simulink model "hiperman_4_2007b_FixPt"  (Simulink 7.2)
settings: Solver=VariableStepDiscrete  SolverMode=SingleTasking  StartTime=0.0  StopTime=inf  RelTol=1e-3
PreLoadFcn:
  | SNR = 17;
  | wl = 16;
undefined symbols (not defined in the file or in its folder): Deinterleaver, get, hiperman_lib, Interleaver
libraries: commutil2 x7, dspobslib x5, commblkcod2 x3, dspsigops x3, commdigbbndam3 x2, commblkintrlv2 x2, dspindex x2, commsequence2 x2, commcnvcod2 x2, commsink2 x2, dspmtrx3 x2, commchan3 x1
CloseFcn:
  | rtwprivate ssgencode ModelCloseRequest hiperman_4_2007b_FixPt
settings Model: Creator=mikem  LastModifiedBy=mdonovan
settings DataIOCC: SaveOutput=off  SaveTime=off
settings OptimizationCC: InlineParams=on  InlineInvariantSignals=on  EnforceIntegerDowncast=off  StateBitsets=on  DataBitsets=on  UseTempVars=on  ZeroExternalMemoryAtStartup=off  ZeroInternalMemoryAtStartup=off  OptimizeModelRefInitCode=on  LifeSpan=1
settings DebuggingCC: AlgebraicLoopMsg=error  SaveWithParameterizedLinksMsg=none  SignalResolutionControl=TryResolveAllWithWarning  MultiTaskDSMMsg=warning  MultiTaskCondExecSysMsg=none  SingleTaskRateTransMsg=error  StrictBusMsg=None  LoggingUnavailableSignals=none
settings HardwareCC: ProdHWDeviceType=Generic->32-bit Embedded Processor  TargetHWDeviceType=32-bit Generic  ProdEqTarget=off
settings RTWCC: SystemTargetFile=ert.tlc  GenCodeOnly=on  TemplateMakefile=ert_default_tmf  Description=Real-Time Workshop Embedded Coder (no auto configuration)  GenerateReport=on  ProcessScript=ert_make_rtw_hook  IncludeHyperlinkInReport=on  LaunchReport=on  IncludeERTFirstTime=on
settings CodeAppCC: IgnoreCustomStorageClasses=off
settings ERTTargetCC: MultiwordLength=2048  GenerateSampleERTMain=on  InlinedParameterPlacement=NonHierarchical  ERTCustomFileTemplate=example_file_process.tlc

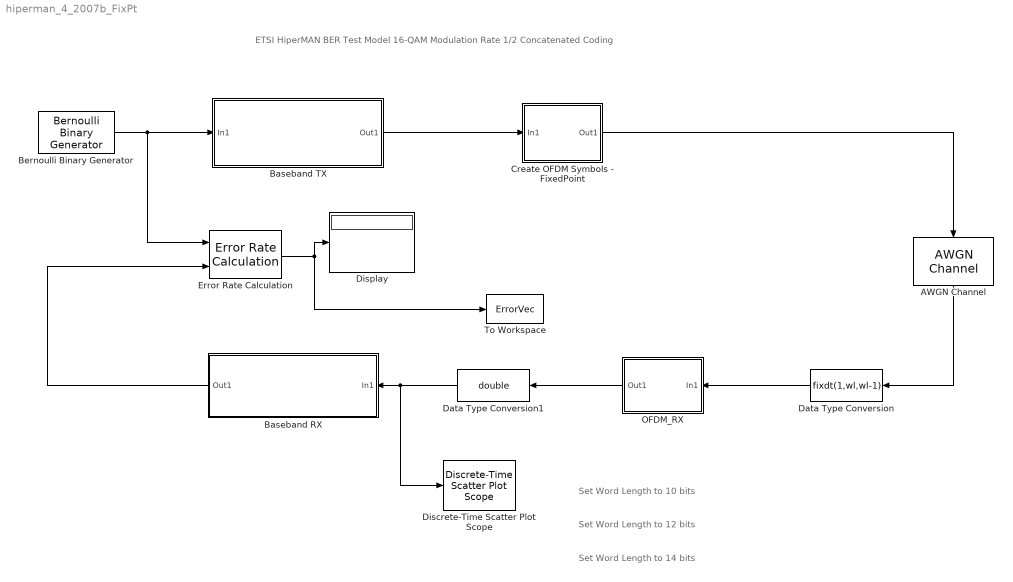
== system hiperman_4_2007b_FixPt ==
  note: ETSI HiperMAN
      | BER Test Model
      | 16-QAM Modulation
      | Rate 1/2 Concatenated Coding
  note: Set Word Length to 12 bits
  note: Set Word Length to 14 bits
  note: Set Word Length to 10 bits
  AWGN Channel : commchan3/AWGN Channel  Orientation=down  SystemSampleTime=-1  seed=67  noiseMode="Signal to noise ratio  (SNR)"  EbNodB=10  EsNodB=10  SNRdB=SNR  bitsPerSym=1  Ps=2/192  Tsym=1  variance=.0004
  Baseband RX : Subsystem  Orientation=left
  Baseband TX : Subsystem
  Bernoulli Binary Generator : commrandsrc2/Bernoulli Binary Generator  DialogController=commDDGCreate  DialogControllerArgs=DataTag3  SystemSampleTime=-1  P=0.5  seed=61  Ts=864/(20e6*3/4*6*32/33*3/4*8/7)/384  frameBased=on  sampPerFrame=384  orient=off  outDataType=double
  Create OFDM Symbols - FixedPoint : Subsystem
      mask Display: disp('Create OFDM\nSymbols');
  Data Type Conversion : DataTypeConversion  Orientation=left  OutDataTypeMode=Specify via dialog  OutDataType=fixdt(1,wl,wl-1)  OutDataTypeStr=fixdt(1,wl,wl-1)
  Data Type Conversion1 : DataTypeConversion  Orientation=left  OutDataTypeMode=double  OutDataType=fixdt(1,16,12)  OutDataTypeStr=double
  Discrete-Time Scatter Plot Scope : commsink2/Discrete-Time Scatter Plot Scope  Tag=ScatterPlot  SystemSampleTime=-1  sampPerSymb=1  offsetEye=0  numTraces=384  numNewFrames=384  LineMarkers=.  LineColors=b  fading=on  render=on  AxisGrid=on  xMin=-1.57265625  xMax=1.47890625  yMin=-1.61953125  yMax=1.43203125  inphaseLabel=In-phase Amplitude  quadratureLabel=Quadrature Amplitude  openScopeAtSimStart=on  FrameNumber=off  FigPos=get(0,'defaultfigureposition');  figTitle=Scatter Plot  numLinesMax=8  block_type_=scatter
  Display : Display
  Error Rate Calculation : commsink2/Error Rate Calculation  N=0  st_delay=0  cp_mode=Entire frame  subframe=[]  PMode=Port  WsName=ErrorVec  RsMode2=off  stop=on  numErr=100  maxBits=1e6
  OFDM_RX : Subsystem  Orientation=left  MinMaxOverflowLogging=MinMaxAndOverflow
      mask Display: disp('Extract Data\nSymbols');
  To Workspace : ToWorkspace  VariableName=ErrorVec  SampleTime=-1  SaveFormat=Array
      settings: MaxDataPoints=1
  wires:
  Create OFDM Symbols - FixedPoint/1(Out1) -> AWGN Channel/1
  AWGN Channel/1 -> Data Type Conversion/1
  Baseband RX/1(Out1) -> Error Rate Calculation/2
  Bernoulli Binary Generator/1 -> Error Rate Calculation/1, Baseband TX/1(In1)
  Baseband TX/1(Out1) -> Create OFDM Symbols - FixedPoint/1(In1)
  Error Rate Calculation/1 -> Display/1, To Workspace/1
  OFDM_RX/1(Out1) -> Data Type Conversion1/1
  Data Type Conversion/1 -> OFDM_RX/1(In1)
  Data Type Conversion1/1 -> Baseband RX/1(In1), Discrete-Time Scatter Plot Scope/1

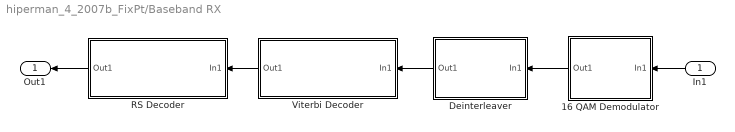
== system hiperman_4_2007b_FixPt/Baseband RX ==
  In1 : Inport  Orientation=left
  16 QAM Demodulator : Subsystem  Orientation=left  AncestorBlock=hiperman_lib/16 QAM Demodulator
      mask init:
      | Ry = ones(4,1)*[+1 +3 -1 -3];
      | Iy = [+1 +3 -3 -1]'*ones(1,4);
      | qamConst = Ry+j*Iy;
      | qamConst = qamConst(:)/sqrt(10);
      | clear Ry Iy;
      mask Display: disp('16 QAM\nDemodulator')
  Deinterleaver : Subsystem  Orientation=left  AncestorBlock=hiperman_lib/Deinterleaver  mask{n1=768, n2=4}
      mask prompts: n1 "Number of coded bits per subchannel:"; n2 "Number of coded bits per subcarrier:"
      mask init:
      | bpc = [192 384 768 1152];
      | pc = [1 2 4 6];
      | Ncbps = bpc(n1);
      | Ncpc = pc(n2);
      | 
      | k = 0:Ncbps-1;
      | mk = (Ncbps/12)*mod(k,12)+floor(k/12);
      | 
      | s = ceil(Ncpc/2);
      | jk = s*floor(mk/s)+mod(mk+Ncbps-floor(12*mk/Ncbps),s);
      | 
      | [x,int_idx] = sort(jk);
      | 
      | clear bpc pc Ncbps Ncpc k mk s jk x
      mask StyleString: popup(192|384|768|1152),popup(1|2|4|6)
      mask Display: disp('Deinterleaver');
  RS Decoder : Subsystem  Orientation=left  AncestorBlock=hiperman_lib/RS Decoder  mask{N=64, K=48}
      mask prompts: N "Input block size (N):"; K "Output block size (K):"
      mask init:
      | % The primitive polynomial is defined over GF(2)
      | primPoly = [1 0 0 0 1 1 1 0 1];  
      | % The generator polynomial is defined over GF(2^8)
      | genPoly = gf([1 1],8);
      | for idx = 1:15
      |     genPoly = conv(genPoly,[1 gf(2,8)^idx]);
      | end
      mask Display: disp('Shortened and Punctured\nReed-Solomon Decoder')
  Viterbi Decoder : Subsystem  Orientation=left  AncestorBlock=hiperman_lib/Viterbi Decoder  mask{ppat=[1 1 0 1]}
      mask prompts: ppat "Puncture pattern:"
      mask Display: disp('Viterbi Decoder\nfor Punctured\nConvolutional Code');
  Out1 : Outport  Orientation=left
  wires:
  16 QAM Demodulator/1(Out1) -> Deinterleaver/1(In1)
  Viterbi Decoder/1(Out1) -> RS Decoder/1(In1)
  Deinterleaver/1(Out1) -> Viterbi Decoder/1(In1)
  In1/1 -> 16 QAM Demodulator/1(In1)
  RS Decoder/1(Out1) -> Out1/1

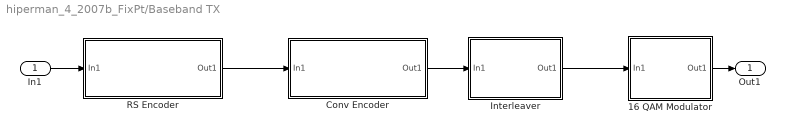
== system hiperman_4_2007b_FixPt/Baseband TX ==
  In1 : Inport
  16 QAM Modulator : Subsystem  AncestorBlock=hiperman_lib/16 QAM Modulator
      mask init:
      | Ry = ones(4,1)*[+1 +3 -1 -3];
      | Iy = [+1 +3 -3 -1]'*ones(1,4);
      | qamConst = Ry+j*Iy;
      | qamConst = qamConst(:)/sqrt(10);
      | clear Ry Iy;
      mask Display: disp('16 QAM\nModulator');
  Conv Encoder : Subsystem  AncestorBlock=hiperman_lib/Conv Encoder  mask{ppat=[1 1 0 1]}
      mask prompts: ppat "Puncture pattern:"
      mask Display: disp('Punctured\nConvolutional Code');
  Interleaver : Subsystem  AncestorBlock=hiperman_lib/Interleaver  mask{n1=768, n2=4}
      mask prompts: n1 "Number of coded bits per subchannel:"; n2 "Number of coded bits per subcarrier:"
      mask init: same as hiperman_4_2007b_FixPt/Baseband RX/Deinterleaver
      mask StyleString: popup(192|384|768|1152),popup(1|2|4|6)
      mask Display: disp('Interleaver')
  RS Encoder : Subsystem  RequirementInfo={'other' 'D:\MBDC2005\ts_102177v010201p.pdf' '#12' 'true' 'Reed-Solomon Coding' '' } %GIDa_a12e56f2_2c6a_45c7_812c_df811bfc8a20  AncestorBlock=hiperman_lib/RS Encoder  mask{N=64, K=48}
      mask prompts: N "Output block size (N):"; K "Input block size (K):"
      mask init: same as hiperman_4_2007b_FixPt/Baseband RX/RS Decoder
      mask Display: disp('Shortened and Punctured\nReed-Solomon Encoder')
  Out1 : Outport
  wires:
  RS Encoder/1(Out1) -> Conv Encoder/1(In1)
  Conv Encoder/1(Out1) -> Interleaver/1(In1)
  Interleaver/1(Out1) -> 16 QAM Modulator/1(In1)
  In1/1 -> RS Encoder/1(In1)
  16 QAM Modulator/1(Out1) -> Out1/1

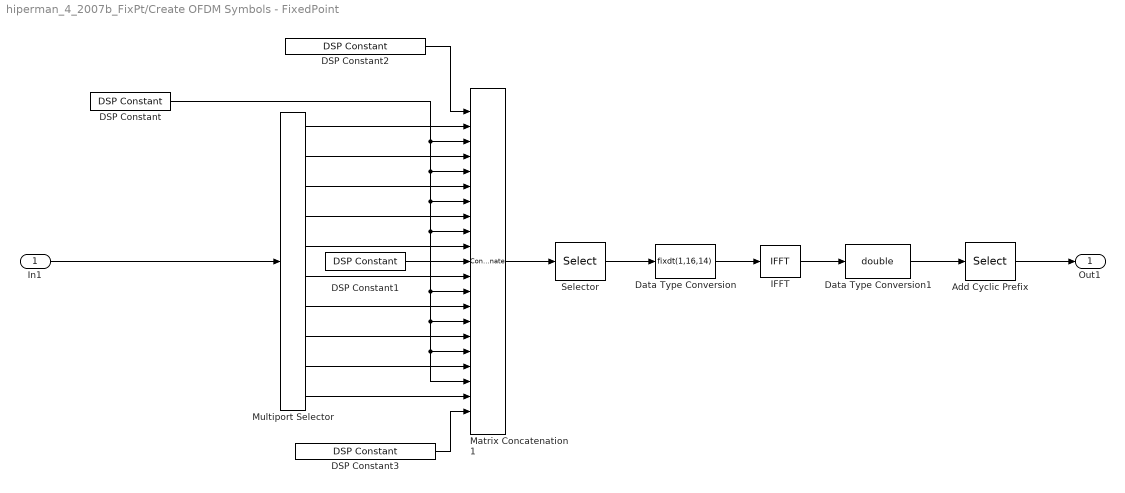
== system hiperman_4_2007b_FixPt/Create OFDM Symbols - FixedPoint ==
  In1 : Inport  OutDataType=sfix(16)  OutScaling=2^0
  Add Cyclic Prefix : Selector  NumberOfDimensions=2  InputPortWidth=3  IndexOptions=Index vector (dialog),Index vector (dialog)  Indices=[251:256 1:256],1  OutputSizes=1,1
  DSP Constant : dspobslib/DSP Constant  SystemSampleTime=-1  Value=complex(1,0)  SampleMode=Discrete  discreteOutput=Frame-based  continuousOutput=Sample-based  sampTime=1  framePeriod=inf  dataType=Inherit from 'Constant value'  isSigned=on  wordLen=16  udDataType=sfix(16)  fracBitsMode=Best precision  numFracBits=15  InterpretAs1D=-inf  Ts=-inf  FramebasedOutput=-inf
  DSP Constant1 : dspobslib/DSP Constant  SystemSampleTime=-1  Value=complex(0,0)  SampleMode=Discrete  discreteOutput=Frame-based  continuousOutput=Sample-based  sampTime=1  framePeriod=inf  dataType=Inherit from 'Constant value'  isSigned=on  wordLen=16  udDataType=sfix(16)  fracBitsMode=Best precision  numFracBits=15  InterpretAs1D=-inf  Ts=-inf  FramebasedOutput=-inf
  DSP Constant2 : dspobslib/DSP Constant  SystemSampleTime=-1  Value=complex(0,0)*ones(28,1)  SampleMode=Discrete  discreteOutput=Frame-based  continuousOutput=Sample-based  sampTime=1  framePeriod=inf  dataType=Inherit from 'Constant value'  isSigned=on  wordLen=16  udDataType=sfix(16)  fracBitsMode=Best precision  numFracBits=15  InterpretAs1D=-inf  Ts=-inf  FramebasedOutput=-inf
  DSP Constant3 : dspobslib/DSP Constant  SystemSampleTime=-1  Value=complex(0,0)*ones(27,1)  SampleMode=Discrete  discreteOutput=Frame-based  continuousOutput=Sample-based  sampTime=1  framePeriod=inf  dataType=Inherit from 'Constant value'  isSigned=on  wordLen=16  udDataType=sfix(16)  fracBitsMode=Best precision  numFracBits=15  InterpretAs1D=-inf  Ts=-inf  FramebasedOutput=-inf
  Data Type Conversion : DataTypeConversion  OutDataTypeMode=Specify via dialog  OutDataType=fixdt(1,16,14)  OutDataTypeStr=fixdt(1,16,14)
  Data Type Conversion1 : DataTypeConversion  OutDataTypeMode=double  OutDataType=fixdt(1,16,12)  OutDataTypeStr=double
  IFFT : dspxfrm3/IFFT  DialogController=dspDDGCreate  DialogControllerArgs=DataTag4  CompMethod=Table lookup  TableOpt=HYBRID  TableOptActive=Speed  BitRevOrder=off  cs_in=off  SkipNorm=on  InheritFFTLength=on  FFTLength=64  mode=Complex  outSamplingMode=Frame based  outputMode=Binary point scaling  outputWordLength=16  outputFracLength=14  accumMode=Binary point scaling  accumWordLength=32  accumFracLength=29  prodOutputMode=Binary point scaling  prodOutputWordLength=32  prodOutputFracLength=30  roundingMode=Floor  overflowMode=off
  Matrix Concatenation1 : Concatenate  NumInputs=21  Mode=Multidimensional array
  Multiport Selector : dspindex/Multiport Selector  rowsOrCols=Rows  idxCellArray={[1:12],[13:36],[37:60],[61:84],[85:96],[97:108],[109:132],[133:156],[157:180],[181:192]}  idxErrMode=Generate Error
  Selector : Selector  InputPortWidth=256  IndexOptions=Index vector (dialog)  Indices=[129:256 1:128]  OutputSizes=1
  Out1 : Outport  OutDataType=sfix(16)  OutScaling=2^0
  wires:
  Data Type Conversion1/1 -> Add Cyclic Prefix/1
  Data Type Conversion/1 -> IFFT/1
  DSP Constant/1 -> Matrix Concatenation1/3, Matrix Concatenation1/5, Matrix Concatenation1/7, Matrix Concatenation1/9, Matrix Concatenation1/13, Matrix Concatenation1/15, Matrix Concatenation1/17, Matrix Concatenation1/19
  Multiport Selector/10 -> Matrix Concatenation1/20
  Multiport Selector/9 -> Matrix Concatenation1/18
  Multiport Selector/8 -> Matrix Concatenation1/16
  Multiport Selector/7 -> Matrix Concatenation1/14
  Multiport Selector/6 -> Matrix Concatenation1/12
  Multiport Selector/5 -> Matrix Concatenation1/10
  Multiport Selector/4 -> Matrix Concatenation1/8
  Multiport Selector/3 -> Matrix Concatenation1/6
  Multiport Selector/2 -> Matrix Concatenation1/4
  Multiport Selector/1 -> Matrix Concatenation1/2
  DSP Constant1/1 -> Matrix Concatenation1/11
  DSP Constant2/1 -> Matrix Concatenation1/1
  DSP Constant3/1 -> Matrix Concatenation1/21
  Matrix Concatenation1/1 -> Selector/1
  In1/1 -> Multiport Selector/1
  Selector/1 -> Data Type Conversion/1
  IFFT/1 -> Data Type Conversion1/1
  Add Cyclic Prefix/1 -> Out1/1

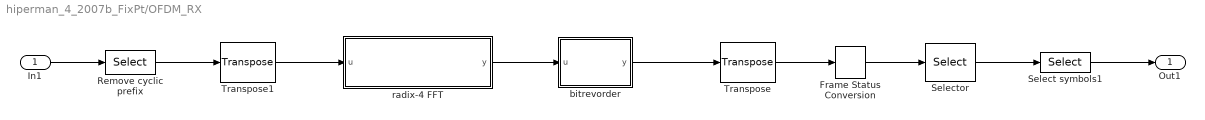
== system hiperman_4_2007b_FixPt/OFDM_RX ==
  In1 : Inport  OutDataType=sfix(16)  OutScaling=2^0
  Frame Status Conversion : dspobslib/Frame Status Conversion  SystemSampleTime=-1  growRefPort=off  outframe=Frame-based
  Remove cyclic prefix : Selector  NumberOfDimensions=2  InputPortWidth=80  IndexOptions=Index vector (dialog),Select all  Indices=[7:262],-1  OutputSizes=1
  Select symbols1 : Selector  NumberOfDimensions=2  InputPortWidth=64  IndexOptions=Index vector (dialog),Select all  Indices=[29:40 42:65 67:90 92:115 117:128 130:141 143:166 168:191 193:216 218:229],-1  OutputSizes=1
  Selector : Selector  InputPortWidth=256  IndexOptions=Index vector (dialog)  Indices=[129:256 1:128]  OutputSizes=1
  Transpose : dspmtrx3/Transpose  SystemSampleTime=-1  Hermitian=off  overflowFlag=off
  Transpose1 : dspmtrx3/Transpose  SystemSampleTime=-1  Hermitian=off  overflowFlag=off
  bitrevorder : Stateflow chart
  radix-4 FFT : Stateflow chart
  Out1 : Outport  OutDataType=sfix(16)  OutScaling=2^0
  wires:
  Transpose1/1 -> radix-4 FFT/1(u)
  Transpose/1 -> Frame Status Conversion/1
  radix-4 FFT/1(y) -> bitrevorder/1(u)
  Remove cyclic prefix/1 -> Transpose1/1
  Frame Status Conversion/1 -> Selector/1
  Selector/1 -> Select symbols1/1
  In1/1 -> Remove cyclic prefix/1
  Select symbols1/1 -> Out1/1
  bitrevorder/1(y) -> Transpose/1

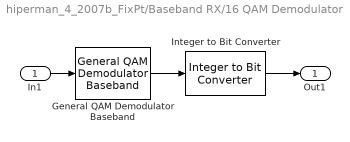
== system hiperman_4_2007b_FixPt/Baseband RX/16 QAM Demodulator ==
  In1 : Inport  OutDataType=sfix(16)  OutScaling=2^0
  General QAM Demodulator Baseband : commdigbbndam3/General QAM Demodulator Baseband  DialogController=commDDGCreate  DialogControllerArgs=DataTag0  SigCon=qamConst  OutType=Integer  DecType=Hard decision  VarSource=Dialog  Variance=1  outDtypeBit=Inherit via internal rule  outDtype=double  roundingMode=Floor  overflowMode=Wrap  sigConstWordLen=16  accum1WordLen=32  accum1FracLen=30  prodInWordLen=32  prodInFracLen=30  prodOutWordLen=32  prodOutFracLen=30  accum2WordLen=32  accum2FracLen=30  accum3WordLen=32  accum3FracLen=30  nsiWordLen=32  nsiFracLen=30  invn0WordLen=16  invn0FracLen=8  outputWordLen=32  outputFracLen=30
  Integer to Bit Converter : commutil2/Integer to Bit Converter  nbits=4  signedInputValues=Unsigned  bitOrder=MSB first  outDtype=Same as input
  Out1 : Outport  OutDataType=sfix(16)  OutScaling=2^0
  wires:
  Integer to Bit Converter/1 -> Out1/1
  General QAM Demodulator Baseband/1 -> Integer to Bit Converter/1
  In1/1 -> General QAM Demodulator Baseband/1

== system hiperman_4_2007b_FixPt/Baseband RX/Deinterleaver ==
  In1 : Inport  OutDataType=sfix(16)  OutScaling=2^0
  General Block Deinterleaver : commblkintrlv2/General Block Deinterleaver  elements=int_idx'
  Out1 : Outport  OutDataType=sfix(16)  OutScaling=2^0
  wires:
  General Block Deinterleaver/1 -> Out1/1
  In1/1 -> General Block Deinterleaver/1

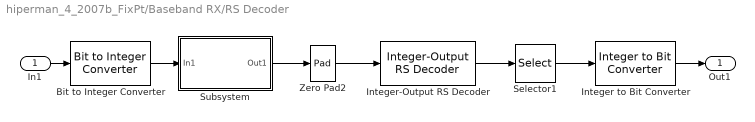
== system hiperman_4_2007b_FixPt/Baseband RX/RS Decoder ==
  In1 : Inport  OutDataType=sfix(16)  OutScaling=2^0
  Bit to Integer Converter : commutil2/Bit to Integer Converter  nbits=8  bitOrder=MSB first  signedOutputValues=Unsigned  outDtype=Same as input  outDtypeSigned=Inherit via internal rule
  Integer to Bit Converter : commutil2/Integer to Bit Converter  nbits=8  signedInputValues=Unsigned  bitOrder=MSB first  outDtype=Same as input
  Integer-Output RS Decoder : commblkcod2/Integer-Output RS Decoder  n=255  k=239  specPrimPoly=on  prPoly=primPoly  specGenPoly=on  genPoly=genPoly  specPuncture=off  punctVec=[ones(2,1); zeros(2,1)]  specErasurePort=off  showNumErr=off
  Selector1 : Selector  InputPortWidth=239  IndexOptions=Index vector (dialog)  Indices=[239-K+1:239]  OutputSizes=1
  Subsystem : Subsystem
      mask Display: disp('Insert Punctured\nParity Bytes');
  Zero Pad2 : dspsigops/Pad  padAlong=Columns  dimsToPad=1  valSrc=Specify via dialog  padVal=0  spec=Output size  padNumOutRowsSpecMethod=User-specified  numOutRows=255  padNumOutColsSpecMethod=User-specified  numOutCols=1  isVarDimsMode=off  padBeginning=0  padEnd=0  outSizeMode=User-specified  outSize=1  padSigAt=Beginning  trunc_flag=None  roundingMode=Floor  overflowMode=off  truncOrWrapMode=Truncate  wrap_flag=None
      settings: AttributesFormatString=\n
  Out1 : Outport  OutDataType=sfix(16)  OutScaling=2^0
  wires:
  Bit to Integer Converter/1 -> Subsystem/1(In1)
  Integer to Bit Converter/1 -> Out1/1
  In1/1 -> Bit to Integer Converter/1
  Selector1/1 -> Integer to Bit Converter/1
  Integer-Output RS Decoder/1 -> Selector1/1
  Zero Pad2/1 -> Integer-Output RS Decoder/1
  Subsystem/1(Out1) -> Zero Pad2/1

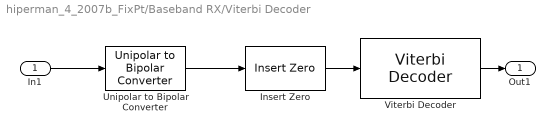
== system hiperman_4_2007b_FixPt/Baseband RX/Viterbi Decoder ==
  In1 : Inport  OutDataType=sfix(16)  OutScaling=2^0
  Insert Zero : commsequence2/Insert Zero  insertZeroVector=ppat(:)
  Unipolar to Bipolar Converter : commutil2/Unipolar to Bipolar Converter  SystemSampleTime=-1  M=2  polarity=Negative  dataType=Same as input
  Viterbi Decoder : commcnvcod2/Viterbi Decoder  DialogController=commDDGCreate  DialogControllerArgs=DataTag1  trellis=poly2trellis(7, [171 133])  isPunctured=off  punctureVector=[1; 1; 0; 1; 0; 1]  erasures=off  dectype=Unquantized  runSigValErrCheck=off  nsdecb=4  smWordLength=16  tbdepth=34  opmode=Truncated  reset=off  outDataType=double
  Out1 : Outport  OutDataType=sfix(16)  OutScaling=2^0
  wires:
  Unipolar to Bipolar Converter/1 -> Insert Zero/1
  Viterbi Decoder/1 -> Out1/1
  In1/1 -> Unipolar to Bipolar Converter/1
  Insert Zero/1 -> Viterbi Decoder/1

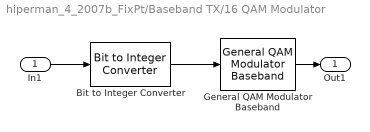
== system hiperman_4_2007b_FixPt/Baseband TX/16 QAM Modulator ==
  In1 : Inport  OutDataType=sfix(16)  OutScaling=2^0
  Bit to Integer Converter : commutil2/Bit to Integer Converter  nbits=4  bitOrder=MSB first  signedOutputValues=Unsigned  outDtype=double  outDtypeSigned=Inherit via internal rule
  General QAM Modulator Baseband : commdigbbndam3/General QAM Modulator Baseband  DialogController=commDDGCreate  DialogControllerArgs=DataTag2  SigCon=qamConst  outDtype=double  outWordLen=16  outUDDataType=sfix(16)  outFracLenMode=Best precision  outFracLen=15
  Out1 : Outport  OutDataType=sfix(16)  OutScaling=2^0
  wires:
  Bit to Integer Converter/1 -> General QAM Modulator Baseband/1
  General QAM Modulator Baseband/1 -> Out1/1
  In1/1 -> Bit to Integer Converter/1

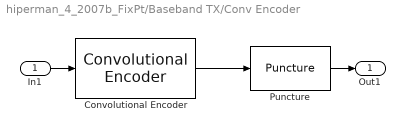
== system hiperman_4_2007b_FixPt/Baseband TX/Conv Encoder ==
  In1 : Inport  OutDataType=sfix(16)  OutScaling=2^0
  Convolutional Encoder : commcnvcod2/Convolutional Encoder  trellis=poly2trellis(7, [171 133])  opMode=Truncated (reset every frame)  hasIniStPort=off  hasFinStPort=off  usePuncVector=off  punctureVector=[1; 1; 0; 1; 0; 1]  reset=Unused parameter value
  Puncture : commsequence2/Puncture  punctureVector=reshape(ppat,numel(ppat),1)
  Out1 : Outport  OutDataType=sfix(16)  OutScaling=2^0
  wires:
  Puncture/1 -> Out1/1
  In1/1 -> Convolutional Encoder/1
  Convolutional Encoder/1 -> Puncture/1

== system hiperman_4_2007b_FixPt/Baseband TX/Interleaver ==
  In1 : Inport  OutDataType=sfix(16)  OutScaling=2^0
  General Block Interleaver : commblkintrlv2/General Block Interleaver  elements=int_idx'
  Out1 : Outport  OutDataType=sfix(16)  OutScaling=2^0
  wires:
  General Block Interleaver/1 -> Out1/1
  In1/1 -> General Block Interleaver/1

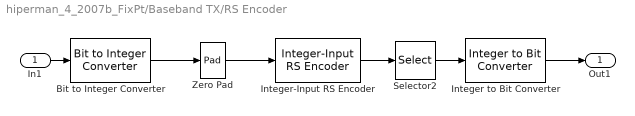
== system hiperman_4_2007b_FixPt/Baseband TX/RS Encoder ==
  In1 : Inport  OutDataType=sfix(16)  OutScaling=2^0
  Bit to Integer Converter : commutil2/Bit to Integer Converter  nbits=8  bitOrder=MSB first  signedOutputValues=Unsigned  outDtype=Same as input  outDtypeSigned=Inherit via internal rule
  Integer to Bit Converter : commutil2/Integer to Bit Converter  nbits=8  signedInputValues=Unsigned  bitOrder=MSB first  outDtype=Same as input
  Integer-Input RS Encoder : commblkcod2/Integer-Input RS Encoder  n=255  k=239  specPrimPoly=on  prPoly=primPoly  specGenPoly=on  genPoly=genPoly  specPuncture=off  punctVec=[ones(2,1); zeros(2,1)]
  Selector2 : Selector  InputPortWidth=255  IndexOptions=Index vector (dialog)  Indices=239+[1:N-K -K+1:0]  OutputSizes=1
  Zero Pad : dspsigops/Pad  padAlong=Columns  dimsToPad=1  valSrc=Specify via dialog  padVal=0  spec=Output size  padNumOutRowsSpecMethod=User-specified  numOutRows=239  padNumOutColsSpecMethod=User-specified  numOutCols=1  isVarDimsMode=off  padBeginning=0  padEnd=0  outSizeMode=User-specified  outSize=1  padSigAt=Beginning  trunc_flag=None  roundingMode=Floor  overflowMode=off  truncOrWrapMode=Truncate  wrap_flag=None
      settings: AttributesFormatString=\n
  Out1 : Outport  OutDataType=sfix(16)  OutScaling=2^0
  wires:
  Integer to Bit Converter/1 -> Out1/1
  Bit to Integer Converter/1 -> Zero Pad/1
  Integer-Input RS Encoder/1 -> Selector2/1
  Zero Pad/1 -> Integer-Input RS Encoder/1
  Selector2/1 -> Integer to Bit Converter/1
  In1/1 -> Bit to Integer Converter/1

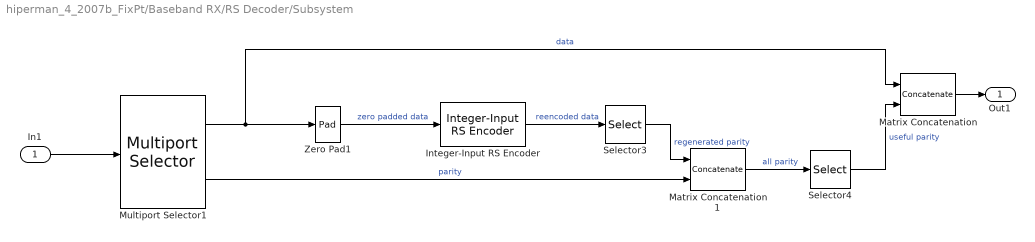
== system hiperman_4_2007b_FixPt/Baseband RX/RS Decoder/Subsystem ==
  In1 : Inport  OutDataType=sfix(16)  OutScaling=2^0
  Integer-Input RS Encoder : commblkcod2/Integer-Input RS Encoder  n=255  k=239  specPrimPoly=on  prPoly=primPoly  specGenPoly=on  genPoly=genPoly  specPuncture=off  punctVec=[ones(2,1); zeros(2,1)]
  Matrix Concatenation : Concatenate  Mode=Multidimensional array
  Matrix Concatenation1 : Concatenate  Mode=Multidimensional array
  Multiport Selector1 : dspindex/Multiport Selector  rowsOrCols=Rows  idxCellArray={[N-K+1:N],[1:N-K]}  idxErrMode=Clip Index
  Selector3 : Selector  InputPortWidth=255  IndexOptions=Index vector (dialog)  Indices=[240:255]  OutputSizes=1
      settings: AttributesFormatString=Elements = %<Elements>\nInput port width = %<InputPortWidth>
  Selector4 : Selector  InputPortWidth=16+N-K  IndexOptions=Index vector (dialog)  Indices=[17:16+N-K N-K+1:16]  OutputSizes=1
      settings: AttributesFormatString=Elements = %<Elements>\nInput port width = %<InputPortWidth>
  Zero Pad1 : dspsigops/Pad  padAlong=Columns  dimsToPad=1  valSrc=Specify via dialog  padVal=0  spec=Output size  padNumOutRowsSpecMethod=User-specified  numOutRows=239  padNumOutColsSpecMethod=User-specified  numOutCols=1  isVarDimsMode=off  padBeginning=0  padEnd=0  outSizeMode=User-specified  outSize=1  padSigAt=Beginning  trunc_flag=None  roundingMode=Floor  overflowMode=off  truncOrWrapMode=Truncate  wrap_flag=None
      settings: AttributesFormatString=\n
  Out1 : Outport  OutDataType=sfix(16)  OutScaling=2^0
  wires:
  Multiport Selector1/2 -> Matrix Concatenation1/2  "parity"
  Selector4/1 -> Matrix Concatenation/2  "useful parity"
  Multiport Selector1/1 -> Matrix Concatenation/1, Zero Pad1/1  "data"
  Matrix Concatenation1/1 -> Selector4/1  "all parity"
  Selector3/1 -> Matrix Concatenation1/1  "regenerated parity"
  Matrix Concatenation/1 -> Out1/1
  In1/1 -> Multiport Selector1/1
  Integer-Input RS Encoder/1 -> Selector3/1  "reencoded data"
  Zero Pad1/1 -> Integer-Input RS Encoder/1  "zero padded data"

== matlab function OFDM_RX/bitrevorder ==
  data: u input double; y output double
function y = bitrev(u)
% This block supports the Embedded MATLAB subset.
% See the help menu for details. 

y = bitrevorder(u);

== matlab function OFDM_RX/radix-4 FFT ==
  data: u input double; y output double
function y = radix4FFT(u)
% This block supports the Embedded MATLAB subset.
% See the help menu for details. 

y = radix4FFT3_FixPtEML(u);
